simulink model "convertToPitchArduino"  (R2022a)
settings: Solver=VariableStepAuto  StartTime=0.0  StopTime=10.0  RelTol=1e-3
libraries: microbitaccellib x1
settings Model: Creator=Ekaterina  LastModifiedBy=Ekaterina

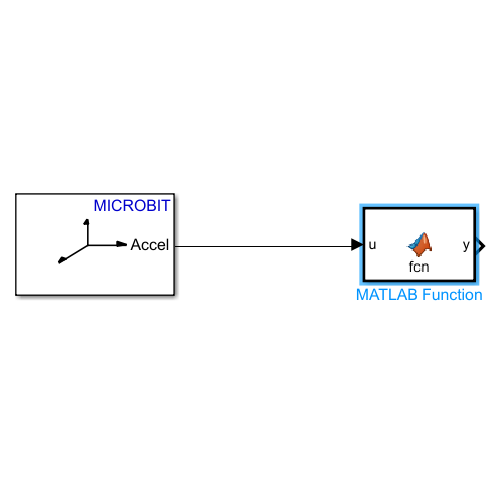
[thumbnail: Simulink's stored preview of the top-level diagram]
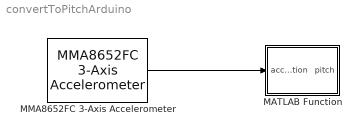
== system convertToPitchArduino ==
  MATLAB Function : MATLAB Function  TreatAsAtomicUnit=on
  MMA8652FC 3-Axis Accelerometer : microbitaccellib/MMA8652FC 3-Axis Accelerometer  ODR=800Hz  Accelfullrange=-4g to +4g  SampleTime=0.1
      settings: SourceProductBaseCode=MICROBIT
  wires:
  MMA8652FC 3-Axis Accelerometer/1 -> MATLAB Function/1(acceleration)

== matlab function convertToPitchArduino/MATLAB Function ==
  data: acceleration input; pitch output
function pitch =convertToPitch (acceleration) 

acceleration_x=acceleration(1);
acceleration_y=acceleration(2);
acceleration_z=acceleration(3);

pitch= atand(acceleration_x/sqrt(acceleration_y^2+acceleration_z^2)); 

end
